simulink model "sf_gfdemo"  (Simulink 7.6)
settings: Solver=ode45  StartTime=0.0  StopTime=10  MaxStep=.01  RelTol=1e-3
settings Model: Creator=The MathWorks Inc.  CovMetricSettings=dcmtr  ExtModeAutoUpdateStatusClock=off
settings OptimizationCC: BooleanDataType=off  InlineInvariantSignals=on  InitFltsAndDblsToZero=on  EfficientMapNaN2IntZero=off
settings DebuggingCC: SaveWithParameterizedLinksMsg=none  SignalResolutionControl=TryResolveAllWithWarning  SolverPrmCheckMsg=none  MultiTaskDSMMsg=warning  MultiTaskCondExecSysMsg=none  StrictBusMsg=None
settings HardwareCC: TargetUnknown=on
settings SFSimCC: SimParseCustomCode=off
settings RTWCC: IncludeERTFirstTime=on
settings GRTTargetCC: TargetFcnLib=ansi_tfl_tmw.mat

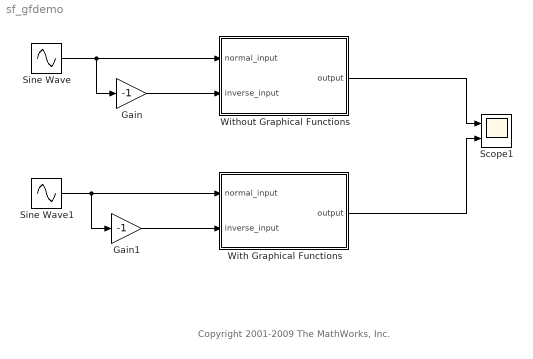
== system sf_gfdemo ==
  note: Copyright 2001-2009 The MathWorks, Inc.
  Gain : Gain  Gain=-1  SaturateOnIntegerOverflow=on  OutDataTypeStr=Inherit: Same as input  ParamDataTypeStr=Inherit: Same as input
  Gain1 : Gain  Gain=-1  SaturateOnIntegerOverflow=on  OutDataTypeStr=Inherit: Same as input  ParamDataTypeStr=Inherit: Same as input
  Scope1 : Scope  NumInputPorts=2
      settings: TimeRange=10  YMin=-0.5~-0.5  YMax=1~1
  Sine Wave : Sin  SampleTime=0
  Sine Wave1 : Sin  SampleTime=0
  With Graphical Functions : Stateflow chart  TreatAsAtomicUnit=on
  Without Graphical Functions : Stateflow chart  TreatAsAtomicUnit=on
  wires:
  Without Graphical Functions/1(output) -> Scope1/1
  With Graphical Functions/1(output) -> Scope1/2
  Sine Wave/1 -> Gain/1, Without Graphical Functions/1(normal_input)
  Gain/1 -> Without Graphical Functions/2(inverse_input)
  Sine Wave1/1 -> Gain1/1, With Graphical Functions/1(normal_input)
  Gain1/1 -> With Graphical Functions/2(inverse_input)

== stateflow chart Without Graphical Functions ==
  state Normal
    (default) -> (junction 5)
    (junction 5) -> (junction 9) [order 1] : [normal_input >0.5]
    (junction 9) -> (junction 10) : {output = 0.5;}
    (junction 5) -> (junction 10) [order 2] : {output=normal_input;}
  state Inverse
    (default) -> (junction 6)
    (junction 6) -> (junction 7) [order 1] : [inverse_input > 0.5]
    (junction 6) -> (junction 8) [order 2] : {output=inverse_input;}
    (junction 7) -> (junction 8) : {output = 0.5;}
  (default) -> Normal
  Normal -> Inverse [order 1] : [normal_input < 0]
  Inverse -> Normal [order 1] : [inverse_input<0]
  Normal -> Normal [order 2]
  Inverse -> Inverse [order 2]
  data: output output double; normal_input input double; inverse_input input double

== stateflow chart With Graphical Functions ==
  state Normal
    (default) -> (junction 33) : {set_output_data(normal_input);}
  state Inverse
    (default) -> (junction 34) : {set_output_data(inverse_input);}
  state set_output_data(input) [function]
    (default) -> (junction 32)
    (junction 32) -> (junction 35) [order 1] : [input>.5]
    (junction 35) -> (junction 36) : {output = 0.5;}
    (junction 32) -> (junction 36) [order 2] : {output = input;}
  (default) -> Normal
  Normal -> Inverse [order 1] : [normal_input < 0]
  Inverse -> Normal [order 1] : [inverse_input<0]
  Normal -> Normal [order 2]
  Inverse -> Inverse [order 2]
  data: input function_input double; output output double; normal_input input double; inverse_input input double
